simulink model "ROSCrtlSimulink"  (R2018b)
settings: Solver=FixedStepAuto  StartTime=0.0  StopTime=inf  FixedStep=0.01  RelTol=1e-3
undefined symbols (not defined in the file or in its folder): Theta, X, Y
libraries: robotlib x3, simulink x1
settings Model: Creator=DwigHT  LastModifiedBy=DwigHT

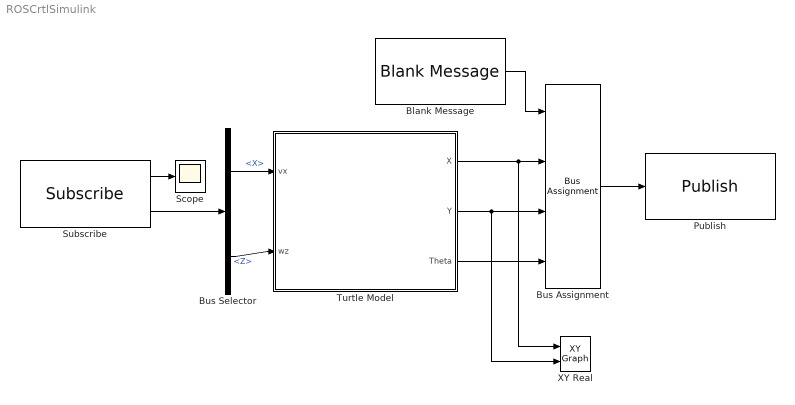
== system ROSCrtlSimulink ==
  Blank Message : robotlib/Blank Message  messageClass=Message  entityType=turtlesim/Pose  messageType=turtlesim/Pose  SampleTime=inf
      settings: SourceProductBaseCode=RO
  Bus Assignment : BusAssignment  AssignedSignals=X,Y,Theta
  Bus Selector : BusSelector  OutputSignals=Linear.X,Angular.Z
  Publish : robotlib/Publish  topicSource=Select from ROS network  topic=/turtle1/pose  messageType=turtlesim/Pose  messageQueueLength=1
      settings: SourceProductBaseCode=RO
  Scope : Scope
  Subscribe : robotlib/Subscribe  topicSource=Select from ROS network  topic=/turtle1/cmd_vel  messageType=geometry_msgs/Twist  sampleTime=-1  messageQueueLength=1
      settings: SourceProductBaseCode=RO
  Turtle Model : Subsystem
  XY Real : simulink/Sinks/XY Graph  xmin=0  xmax=11  ymin=0  ymax=11  st=-1
  wires:
  Bus Selector/1 -> Turtle Model/1(vx)  "<X>"
  Bus Selector/2 -> Turtle Model/2(wz)  "<Z>"
  Blank Message/1 -> Bus Assignment/1
  Turtle Model/2(Y) -> XY Real/2, Bus Assignment/3
  Turtle Model/1(X) -> XY Real/1, Bus Assignment/2
  Turtle Model/3(Theta) -> Bus Assignment/4
  Bus Assignment/1 -> Publish/1
  Subscribe/2 -> Bus Selector/1
  Subscribe/1 -> Scope/1

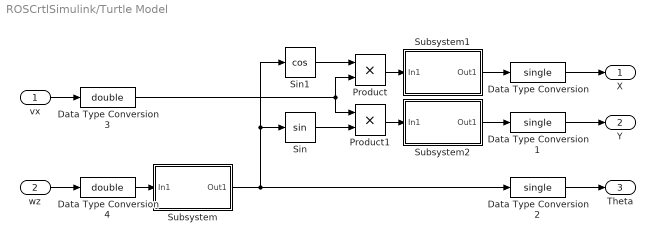
== system ROSCrtlSimulink/Turtle Model ==
  vx : Inport
  wz : Inport  Port=2
  Data Type Conversion : DataTypeConversion  OutDataTypeStr=single
  Data Type Conversion1 : DataTypeConversion  OutDataTypeStr=single
  Data Type Conversion2 : DataTypeConversion  OutDataTypeStr=single
  Data Type Conversion3 : DataTypeConversion  OutDataTypeStr=double
  Data Type Conversion4 : DataTypeConversion  OutDataTypeStr=double
  Product : Product
  Product1 : Product
  Sin : Trigonometry
  Sin1 : Trigonometry  Operator=cos
  Subsystem : Subsystem
  Subsystem1 : Subsystem
  Subsystem2 : Subsystem
  X : Outport
  Y : Outport  Port=2
  Theta : Outport  Port=3
  wires:
  Product1/1 -> Subsystem2/1(In1)
  Subsystem2/1(Out1) -> Data Type Conversion1/1
  Sin1/1 -> Product/1
  Subsystem1/1(Out1) -> Data Type Conversion/1
  vx/1 -> Data Type Conversion3/1
  Product/1 -> Subsystem1/1(In1)
  Subsystem/1(Out1) -> Data Type Conversion2/1, Sin/1, Sin1/1
  Sin/1 -> Product1/2
  wz/1 -> Data Type Conversion4/1
  Data Type Conversion/1 -> X/1
  Data Type Conversion1/1 -> Y/1
  Data Type Conversion2/1 -> Theta/1
  Data Type Conversion3/1 -> Product/2, Product1/1
  Data Type Conversion4/1 -> Subsystem/1(In1)

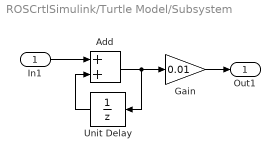
== system ROSCrtlSimulink/Turtle Model/Subsystem ==
  In1 : Inport
  Add : Sum
  Gain : Gain  Gain=0.01
  Unit Delay : UnitDelay  SampleTime=0.01
  Out1 : Outport
  wires:
  Unit Delay/1 -> Add/2
  Add/1 -> Gain/1, Unit Delay/1
  Gain/1 -> Out1/1
  In1/1 -> Add/1

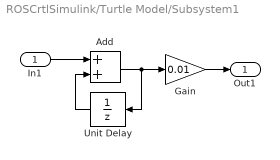
== system ROSCrtlSimulink/Turtle Model/Subsystem1 ==
  In1 : Inport
  Add : Sum
  Gain : Gain  Gain=0.01
  Unit Delay : UnitDelay  InitialCondition=555  SampleTime=0.01
  Out1 : Outport
  wires:
  In1/1 -> Add/1
  Gain/1 -> Out1/1
  Add/1 -> Unit Delay/1, Gain/1
  Unit Delay/1 -> Add/2

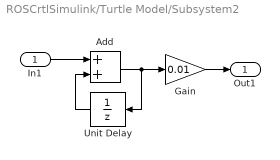
== system ROSCrtlSimulink/Turtle Model/Subsystem2 ==
  In1 : Inport
  Add : Sum
  Gain : Gain  Gain=0.01
  Unit Delay : UnitDelay  InitialCondition=555  SampleTime=0.01
  Out1 : Outport
  wires:
  Unit Delay/1 -> Add/2
  Add/1 -> Gain/1, Unit Delay/1
  Gain/1 -> Out1/1
  In1/1 -> Add/1
